simulink model "1"  (R2022a)
settings: Solver=VariableStepAuto  StartTime=0.0  StopTime=200  RelTol=1e-3
undefined symbols (not defined in the file or in its folder): a1, a2, a3, b, m
libraries: fuzblock x1, slpidlib x1
settings Model: Creator=steli  LastModifiedBy=steli

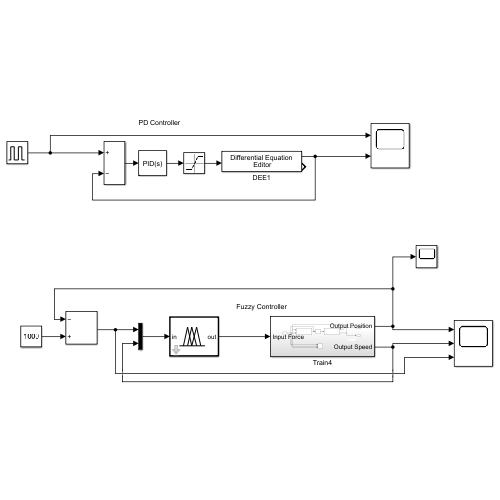
[thumbnail: Simulink's stored preview of the top-level diagram]
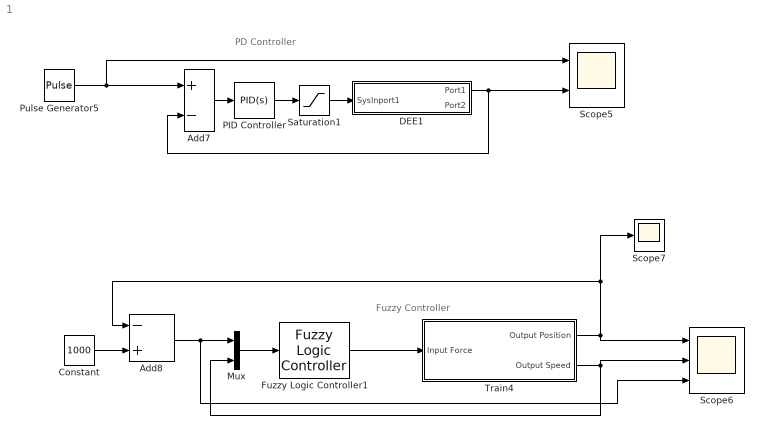
== system 1 ==
  note: PD Controller
  note: Fuzzy Controller
  Add7 : Sum  Inputs=+-
  Add8 : Sum  Inputs=-+
  Constant : Constant  Value=1000
  DEE1 : Subsystem  mask(Differential Equation Editor (DEE)){}
      settings: OpenFcn=diffeqed
      mask Display: disp('Differential Equation\n Editor')
  Fuzzy Logic Controller1 : fuzblock/Fuzzy Logic  Controller  FIS='FuzzyControllerTesting.fis'  OutputSampleNumber=101  DataType=double  FuzzifiedInputs=off  RuleFiringStrengths=off  RuleOutputs=off  AggregatedOutputs=off  SimulateUsing=Interpreted execution  OutOfRangeInputValueMessage=warning  NoRuleFiredMessage=warning  EmptyOutputFuzzySetMessage=warning
  Mux : Mux  Inputs=2
  PID Controller : slpidlib/PID Controller  Controller=PID  Form=Parallel  TimeDomain=Continuous-time  UseExternalTs=off  SampleTime=-1  IntegratorMethod=Forward Euler  FilterMethod=Forward Euler  ControllerParametersSource=internal  P=0.01  I=0  UseKiTs=off  D=0.1  N=100  UseFilter=on  TunerSelectOption=Transfer Function Based (PID Tuner App)  InitialConditionSource=internal  InitialConditionForIntegrator=0  InitialConditionForFilter=0  DifferentiatorICPrevScaledInput=0  ExternalReset=none  TrackingMode=off  Kt=1  LimitOutput=off  SatLimitsSource=internal  UpperSaturationLimit=inf  LowerSaturationLimit=-inf  LinearizeAsGain=on  AntiWindupMode=none  Kb=1  POutMin=[]  POutMax=[]  IOutMin=[]  IOutMax=[]  DOutMin=[]  DOutMax=[]  NOutMin=[]  NOutMax=[]  SumOutMin=[]  SumOutMax=[]  SaturationOutMin=[]  SaturationOutMax=[]  PParamMin=[]  PParamMax=[]  IParamMin=[]  IParamMax=[]  DParamMin=[]  DParamMax=[]  NParamMin=[]  NParamMax=[]  KbParamMin=[]  KbParamMax=[]  KtParamMin=[]  KtParamMax=[]  KbOutMin=[]  KbOutMax=[]  KtOutMin=[]  KtOutMax=[]  IntegratorOutMin=[]  IntegratorOutMax=[]  FilterOutMin=[]  FilterOutMax=[]  SumI1OutMin=[]  SumI1OutMax=[]  SumI2OutMin=[]  SumI2OutMax=[]  SumI3OutMin=[]  SumI3OutMax=[]  SumI4OutMin=[]  SumI4OutMax=[]  SumDOutMin=[]  SumDOutMax=[]  DifferentiatorOutMin=[]  DifferentiatorOutMax=[]  FilterDiffOutCoefMin=[]  FilterDiffOutCoefMax=[]  ReciprocalOutMin=[]  ReciprocalOutMax=[]  SumDenOutMin=[]  SumDenOutMax=[]  SumNumOutMin=[]  SumNumOutMax=[]  DivideOutMin=[]  DivideOutMax=[]  UdiffTsProdOutMin=[]  UdiffTsProdOutMax=[]  NTsProdOutMin=[]  NTsProdOutMax=[]  UintegralTsProdOutMin=[]  UintegralTsProdOutMax=[]  UngainTsProdOutMin=[]  UngainTsProdOutMax=[]  IntegratorContinuousStateAttributes=''  IntegratorStateMustResolveToSignalObject=off  IntegratorRTWStateStorageClass=Auto  FilterContinuousStateAttributes=''  FilterStateMustResolveToSignalObject=off  FilterRTWStateStorageClass=Auto  ParallelPVariant=InternalParameters  IdealPVariant=Disabled  IVariant=InternalParameters  DVariant=InternalParameters  IntegratorVariant=Continuous  SatVariant=Disabled  AWVariant=Passthrough  PCopyVariant=Disabled  TRVariant=Disabled  FdbkBlocksVariant=Forward  IdealPFdbkVariant=Disabled  SatFdbkVariant=Disabled  DerivativeFilterVariant=ContFilter  NVariant=InternalParameters  NCopyVariant=Disabled  FilterICVariant=InternalICsFilter  IntegratorICVariant=InternalICs  ExternalResetVariant=Disabled  TRSumVariant=Passthrough  SumFdbkVariant=Disabled  SumVariant=Sum_PID  TsampFilterVariant=InternalTs  TsampNgainVariant=Passthrough  TsampIntegralVariant=Passthrough  ExternalSaturationOutDataTypeStr=Inherit: Same as second input  aMode=0
  Pulse Generator5 : DiscretePulseGenerator  PulseType=Time based  Amplitude=10  Period=500  PulseWidth=40
  Saturation1 : Saturate
  Scope5 : Scope  NumInputPorts=2
  Scope6 : Scope  NumInputPorts=3
  Scope7 : Scope
  Train4 : Subsystem
  wires:
  Mux/1 -> Fuzzy Logic Controller1/1
  Add8/1 -> Scope6/3, Mux/1
  Pulse Generator5/1 -> Scope5/1, Add7/1
  Train4/2(Output Speed) -> Mux/2, Scope6/2
  Constant/1 -> Add8/2
  Fuzzy Logic Controller1/1 -> Train4/1(Input Force)
  Train4/1(Output Position) -> Scope7/1, Add8/1, Scope6/1
  PID Controller/1 -> Saturation1/1
  Saturation1/1 -> DEE1/1(SysInport1)
  Add7/1 -> PID Controller/1
  DEE1/1(Port1) -> Scope5/2, Add7/2

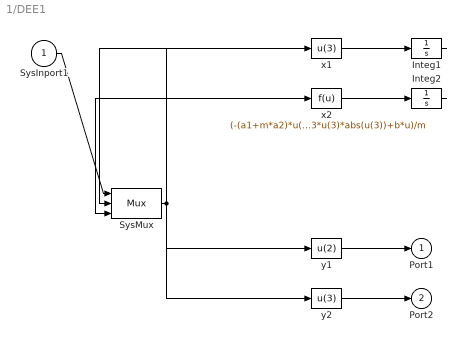
== system 1/DEE1 ==
  SysInport1 : Inport
  Integ1 : Integrator
  Integ2 : Integrator
  SysMux : Mux  Inputs=3
  x1 : Fcn  Expr=u(3)
  x2 : Fcn  Expr=(-(a1+m*a2)*u(3)-a3*u(3)*abs(u(3))+b*u)/m
  y1 : Fcn  Expr=u(2)
  y2 : Fcn  Expr=u(3)
  Port1 : Outport
  Port2 : Outport  Port=2
  wires:
  SysInport1/1 -> SysMux/1
  SysMux/1 -> x1/1, x2/1, y1/1, y2/1
  x1/1 -> Integ1/1
  Integ1/1 -> SysMux/2
  x2/1 -> Integ2/1
  Integ2/1 -> SysMux/3
  y1/1 -> Port1/1
  y2/1 -> Port2/1

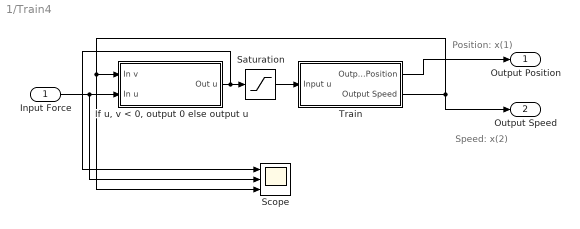
== system 1/Train4 ==
  note: Speed: x(2)
  note: Position: x(1)
  Input Force : Inport
  "If u, v < 0, output 0 else output u" : Subsystem
  Saturation : Saturate  UpperLimit=1  LowerLimit=-1
  Scope : Scope  NumInputPorts=3
  Train : Subsystem
  Output Position : Outport
  Output Speed : Outport  Port=2
  wires:
  Input Force/1 -> "If u, v < 0, output 0 else output u"/2(In u), Scope/2
  Train/1(Output Position) -> Output Position/1
  Train/2(Output Speed) -> Output Speed/1, Scope/3, "If u, v < 0, output 0 else output u"/1(In v)
  "If u, v < 0, output 0 else output u"/1(Out u) -> Saturation/1, Scope/1
  Saturation/1 -> Train/1(Input u)

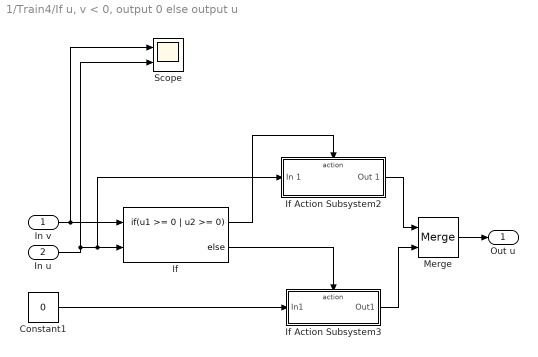
== system 1/Train4/If u, v < 0, output 0 else output u ==
  In v : Inport
  In u : Inport  Port=2
  Constant1 : Constant  Value=0
  If : If  NumInputs=2  IfExpression=u1 >= 0 | u2 >= 0
  If Action Subsystem2 : Subsystem  TreatAsAtomicUnit=on
  If Action Subsystem3 : Subsystem  TreatAsAtomicUnit=on
  Merge : Merge
  Scope : Scope  NumInputPorts=2
  Out u : Outport
  wires:
  If/1 -> If Action Subsystem2/Action
  In v/1 -> Scope/1, If/1
  Constant1/1 -> If Action Subsystem3/1(In1)
  Merge/1 -> Out u/1
  If Action Subsystem3/1(Out1) -> Merge/2
  If Action Subsystem2/1(Out 1) -> Merge/1
  In u/1 -> Scope/2, If Action Subsystem2/1(In 1), If/2
  If/2 -> If Action Subsystem3/Action

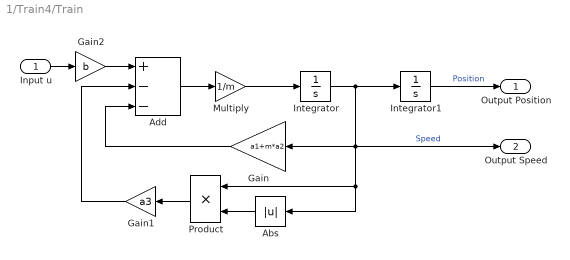
== system 1/Train4/Train ==
  Input u : Inport
  Abs : Abs  SaturateOnIntegerOverflow=off
  Add : Sum  Inputs=+--
  Gain : Gain  Gain=a1+m*a2
  Gain1 : Gain  Gain=a3
  Gain2 : Gain  Gain=b
  Integrator : Integrator
  Integrator1 : Integrator
  Multiply : Gain  Gain=1/m
  Product : Product
  Output Position : Outport
  Output Speed : Outport  Port=2
  wires:
  Multiply/1 -> Integrator/1
  Input u/1 -> Gain2/1
  Add/1 -> Multiply/1
  Integrator/1 -> Abs/1, Product/1, Output Speed/1, Gain/1, Integrator1/1  "Speed"
  Integrator1/1 -> Output Position/1  "Position"
  Gain/1 -> Add/3
  Abs/1 -> Product/2
  Product/1 -> Gain1/1
  Gain1/1 -> Add/2
  Gain2/1 -> Add/1

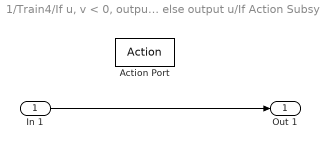
== system 1/Train4/If u, v < 0, output 0 else output u/If Action Subsystem2 ==
  In 1 : Inport
  Action Port : ActionPort  ActionPortLabel=if(u1 >= 0 | u2 >= 0)
  Out 1 : Outport
  wires:
  In 1/1 -> Out 1/1

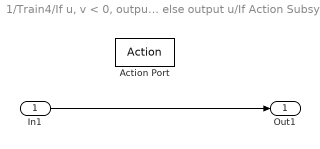
== system 1/Train4/If u, v < 0, output 0 else output u/If Action Subsystem3 ==
  In1 : Inport
  Action Port : ActionPort  ActionPortLabel=else
  Out1 : Outport
  wires:
  In1/1 -> Out1/1
